simulink model "Tega0x2DNew"  (R2023b)
settings: Solver=VariableStepAuto  StartTime=0.0  StopTime=5  RelTol=1e-3
undefined symbols (not defined in the file): Ion, Lithium
libraries: spsSeriesRLCBranchLib x6, spsUniversalBridgeLib x2, spsThreePhaseParallelRLCLoadLib x1, spsBatteryLib x1, spsCurrentMeasurementLib x1, spsDieselMotorModel x1, spsDiodeLib x1, spsAC1AExcitationSystemLib x1, spsAC4AExcitationSystemLib x1, spsAC5AExcitationSystemLib x1, spsDC1AExcitationSystemLib x1, spsDC2AExcitationSystemLib x1
settings Model: Creator=HP  LastModifiedBy=HP

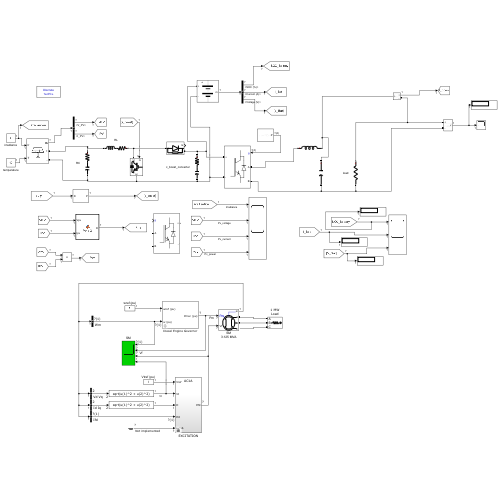
[thumbnail: Simulink's stored preview of the top-level diagram]
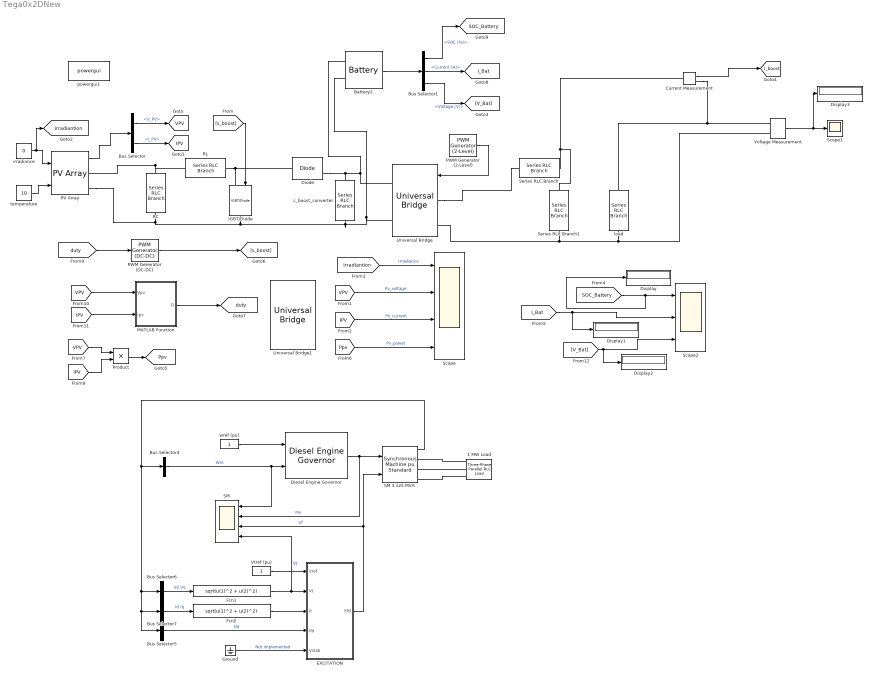
== system Tega0x2DNew ==
  1 MW Load : spsThreePhaseParallelRLCLoadLib/Three-Phase Parallel RLC Load  LConnTagsString=A|B|C  Configuration=Y (grounded)  NominalVoltage=2400  Vabc=[1e3 1e3 1e3]  Vabcp=[1e3 1e3 1e3]  NominalFrequency=60  UnbalancedPower=off  ActivePower=1e+006  InductivePower=0  CapacitivePower=0  Pabc=[10e3 9e3 11e3]  QLabc=[100 90 110]  QCabc=[100 90 110]  Pabcp=[10e3 9e3 11e3]  QLabcp=[100 90 110]  QCabcp=[100 90 110]  Measurements=None  LoadType=constant Z
  Battery2 : spsBatteryLib/Battery  BatType=Lithium-Ion  ShowTempParam=off  ThermalPreset=no  ShowAgeParam=off  NomV=12  NomQ=100  SOC=45  Batt_Tr=1  PresetModel=on  MaxQ=100  MinV=9  FullV=13.9678  Dis_rate=43.4783  R=0.0012  Normal_OP=90.4348  expZone="[12.9646      4.91304]"  current=[6.5 13 32.5]  Units=Time  Tci=20  NomT=20  T2=-30  MaxQ2=4.8  FullV2=7.1  Normal_OP2=5.655  expZone2="[6.58           1]"  Rca=0.6  ti=2000  Dp=0  Neq0=0  Tsim=1e6  Ta1=25  Qeol=5.4*0.9  Reol=0.013333*1.2  Char_age=[2.3478, 3]  Dis_age=[2.3478, 10]  N1=1500  N2=10500  N3=1000  N4=1400  Ta2=45  N5=950
  Bus Selector : BusSelector  OutputSignals=V_PV,I_PV
  Bus Selector1 : BusSelector  OutputSignals=SOC (%),Current (A),Voltage (V)
  Bus Selector4 : BusSelector  OutputSignals="Mechanical.Rotor speed  wm  (pu)"  OutputAsBus=on
  Bus Selector5 : BusSelector  OutputSignals="dq0 components.Field current  ifd (pu)"  OutputAsBus=on
  Bus Selector6 : BusSelector  OutputSignals="dq0 components.Stator voltage  vd (pu),dq0 components.Stator voltage  vq (pu)"  OutputAsBus=on
  Bus Selector7 : BusSelector  OutputSignals="dq0 components.Stator current  id (pu),dq0 components.Stator current  iq (pu)"  OutputAsBus=on
  Current Measurement : spsCurrentMeasurementLib/Current Measurement  PhasorSimulation=off  OutputType=Complex  PSBequivalent=0
  Diesel Engine Governor : spsDieselMotorModel/Diesel Engine Governor  K=40  Tr=[0.01 0.02 0.2]  Ta=[0.25 0.009 0.0384]  Tlim=[0 1.1]  Td=0.024  Pm0=0
  Diode : spsDiodeLib/Diode  Ron=0.001  Lon=0  Vf=0.8  IC=0  UseSnubber=0  Rs=500  Cs=250e-9  Measurements=on
  Display{,1..3} (4 alike) : Display
  EXCITATION : Subsystem  Variant=on  VariantControlMode=label  LabelModeActiveChoice=Variant1
      settings: AttributesFormatString=%<BlockChoice>
  Fcn1 : Fcn  Expr=sqrt(u(1)^2 + u(2)^2)
  Fcn2 : Fcn  Expr=sqrt(u(1)^2 + u(2)^2)
  Ground : Ground
  IGBT/Diode : spsIGBTDiodeLib/IGBT//Diode  Ron=1e-3  Rs=1e5  Cs=inf  Measurements=off
  MATLAB Function : MATLAB Function  TreatAsAtomicUnit=on
  PV Array : spsPVArrayLib/PV Array  Npar=6  Nser=2  PlotType=array @ 1000 W/m2 & specified temperatures  S_vec="[ 1000  500  100 ]"  Temp_C_vec="[ 45 25  ]"  ModuleName=User-defined  PlotWhenSelected=off  Pm=380.16  Ncell=72  Voc=48.7  Isc=9.98  Vm=39.6  Im=9.6  beta_Voc_pc=-0.32  alpha_Isc_pc=0.05  beta_Voc=-0.15584  alpha_Isc=0.00499  IL=10.0548  I0=7.7106e-11  nI=1.0287  Rsh=2826.5806  Rs=0.35496  RobustModel=off  RobustCellTemperature=313.3991  BAL=on  Tc=1e-6  Tfilter=5e-5
  PWM Generator (2-Level) : spsPWMGenerator2LevelLib/PWM Generator (2-Level)  ModulatorType=Single-phase full-bridge (4 pulses)  ModulatorMode=Unsynchronized  Fc=27*60  Pc=90  nF=27  MinMax="[ -1  1 ]"  SamplingTechnique=Natural  ModulatingSignals=on  m=0.8  Freq=60  Phase=0  Ts=0  ShowCarrierOutport=off
  PWM Generator (DC-DC) : spsPWMGeneratorDCDCLib/PWM Generator (DC-DC)  Fsw=5000  Ts=10e-6
  Product : Product
  RC : spsSeriesRLCBranchLib/Series RLC Branch  LConnTagsString=__new0  RConnTagsString=__new0  BranchType=RC  Resistance=1e-4  Inductance=1e-3  SetiL0=off  InitialCurrent=0  Capacitance=100e-6  Setx0=off  InitialVoltage=0  Measurements=None
  RL : spsSeriesRLCBranchLib/Series RLC Branch  LConnTagsString=__new0  RConnTagsString=__new0  BranchType=RL  Resistance=0.1  Inductance=5e-3  SetiL0=off  InitialCurrent=0  Capacitance=100e-6  Setx0=off  InitialVoltage=0  Measurements=None
  SM : Scope  NumInputPorts=4
  SM 3.125 MVA : spsSynchronousMachinepuStandardLib/Synchronous Machine pu Standard  PresetModel=No  MechanicalLoad=Mechanical power Pm  ShowDetailedParameters=on  RotorType=Salient-pole  Units=per unit standard parameters  MeasurementBus=off  NominalParameters="[ 3.125e6  2400  60]"  Reactances1=[ 31 32 33 34 35 36 37 ]  Reactances2=[ 1.56, 0.296, 0.177, 1.06, 0.177, 0.052 ]  dAxisTimeConstants=Short-circuit  qAxisTimeConstants=Open-circuit  TimeConstants1=[]  TimeConstants2=[]  TimeConstants3=[]  TimeConstants4=[]  TimeConstants5=[ 3.7, 0.05, 0.05 ]  TimeConstants6=[ 8.0, 0.03, 0.3371, 0.0295 ]  TimeConstants7=[0.024 0.006 0.006]  TimeConstants8=[]  StatorResistance=0.0036  Mechanical="[ 1.07  0 2]"  PolePairs=2  InitialConditions=[0 0 0 0 0 0 0 0 1]  SetSaturation=off  Saturation=[0.211 0.418 1.0 1.25 1.72 3.35 ;0.25 0.50 1.0 1.1 1.2 1.4]  LoadFlowParameters=[1 0 0 0]  TsPowergui=0  TsBlock=-1  IterativeModel=Trapezoidal non iterative  IterativeDiscreteModel=Trapezoidal non iterative  BusType=PV  Pref=0  Qref=0  Qmin=-Inf  Qmax=Inf  PLF=0  QLF=0
  Scope : Scope  NumInputPorts=4
  Scope1 : Scope
  Scope2 : Scope  NumInputPorts=3
  Series RLC Branch : spsSeriesRLCBranchLib/Series RLC Branch  LConnTagsString=__new0  RConnTagsString=__new0  BranchType=L  Resistance=1  Inductance=0.02  SetiL0=off  InitialCurrent=0  Capacitance=1e-6  Setx0=off  InitialVoltage=0  Measurements=None
  Series RLC Branch1 : spsSeriesRLCBranchLib/Series RLC Branch  LConnTagsString=__new0  RConnTagsString=__new0  BranchType=C  Resistance=1  Inductance=1e-3  SetiL0=off  InitialCurrent=0  Capacitance=0.006  Setx0=off  InitialVoltage=0  Measurements=None
  Universal Bridge : spsUniversalBridgeLib/Universal Bridge  Arms=2  SnubberResistance=1e5  SnubberCapacitance=inf  Device=IGBT / Diodes  Ron=1e-3  Lon=0  ForwardVoltages="[  0  0  ]"  ForwardVoltage=0  GTOparameters=[ 10e-6 , 20e-6 ]  IGBTparameters=[ 1e-6 , 2e-6 ]  Measurements=None  Measurements_2=None  converterType=Rectifier
  Universal Bridge1 : spsUniversalBridgeLib/Universal Bridge  Arms=2  SnubberResistance=1e5  SnubberCapacitance=inf  Device=IGBT / Diodes  Ron=1e-3  Lon=0  ForwardVoltages="[  0  0  ]"  ForwardVoltage=0  GTOparameters=[ 10e-6 , 20e-6 ]  IGBTparameters=[ 1e-6 , 2e-6 ]  Measurements=None  Measurements_2=None  converterType=Rectifier
  Voltage Measurement : spsVoltageMeasurementLib/Voltage Measurement  PhasorSimulation=off  OutputType=Complex  PSBequivalent=0
  "Vtref (pu) " : Constant
  c_boost_converter : spsSeriesRLCBranchLib/Series RLC Branch  LConnTagsString=__new0  RConnTagsString=__new0  BranchType=RC  Resistance=1e-4  Inductance=1e-3  SetiL0=off  InitialCurrent=0  Capacitance=3300e-6  Setx0=off  InitialVoltage=0  Measurements=None
  irradiance : Constant  Value=0
  load : spsSeriesRLCBranchLib/Series RLC Branch  LConnTagsString=__new0  RConnTagsString=__new0  BranchType=R  Resistance=10  Inductance=1e-3  SetiL0=off  InitialCurrent=0  Capacitance=3300e-6  Setx0=off  InitialVoltage=0  Measurements=None
  powergui1 : spspowerguiLib/powergui  Priority=1  SimulationMode=Discrete  SampleTime=1e-05  frequency=60  Iterations=50  frequencyindice=0  Pbase=100e6  ErrMax=1e-4  UnitsV=kV  UnitsW=MW  buscounter=0  FunctionMessages=off  echomessages=off  EnableUseOfTLC=off  CurrentSourceSwitches=off  DisableSnubberDevices=off  DisableRonSwitches=off  DisableVfSwitches=off  DisplayEquations=off  AutomaticDiscreteSolvers=off  SolverType=Tustin/Backward Euler (TBE)  Interpol=off  ExternalGateDelay=off  methode=off  Ts=100  x0status=blocks  SPID=on  SwTol=0  HookPort=off  NonlinearTolerance=1e-4  nMaxIteration=100  ContinueOnMaxIteration=off  RestoreLinks=warning  ResistiveCurrentMeasurement=off  Frange=[0:2:500]  Ylog=off  Xlog=on  ShowGrid=off  save=off  variable=ZData  structure=0  ZoomFFT=off  StartTime=0.0  cycles=1  DisplayStyle=1  fundamental=60  FreqAxis=off  MaxFrequency=1000  frequencyindicesteady=1  RmsSteady=1  display=off
  temperature : Constant  Value=10
  wref (pu) : Constant
  tag scope: IPV=global, I_Bat=global, I_boost=global, Ppv=global, SOC_Battery=global, VPV=global, duty=global, irradiantion=global
  wires:
  PV Array/1 -> Bus Selector/1
  Bus Selector/1 -> [VPV]  "<V_PV>"
  Bus Selector/2 -> [IPV]  "<I_PV>"
  temperature/1 -> PV Array/2
  irradiance/1 -> [irradiantion], PV Array/1
  [s_boost] -> IGBT/Diode/1
  Voltage Measurement/1 -> Display3/1, Scope1/1
  Current Measurement/1 -> [I_boost]
  [irradiantion] -> Scope/1  "Irradiance"
  [VPV] -> Scope/2  "Pv_voltage"
  [IPV] -> Scope/3  "Pv_current"
  Product/1 -> [Ppv]
  [VPV] -> Product/1
  [IPV] -> Product/2
  PWM Generator (DC-DC)/1 -> [s_boost]
  [duty] -> PWM Generator (DC-DC)/1
  [VPV] -> MATLAB Function/1(Vpv)
  [IPV] -> MATLAB Function/2(Ipv)
  MATLAB Function/1(D) -> [duty]
  PWM Generator (2-Level)/1 -> Universal Bridge/1
  [Ppv] -> Scope/4  "Pv_power"
  Battery2/1 -> Bus Selector1/1
  Bus Selector1/1 -> [SOC_Battery]  "<SOC (%)>"
  Bus Selector1/2 -> [I_Bat]  "<Current (A)>"
  Bus Selector1/3 -> [V_Bat]  "<Voltage (V)>"
  [I_Bat] -> Display1/1, Scope2/2
  [V_Bat] -> Display2/1, Scope2/3
  [SOC_Battery] -> Display/1, Scope2/1
  SM 3.125 MVA/1 -> Bus Selector4/1, Bus Selector6/1, Bus Selector7/1, Bus Selector5/1
  Fcn1/1 -> SM/4, EXCITATION/2(Vt)  "Vt"
  EXCITATION/1(Efd) -> SM/3, SM 3.125 MVA/2  "Vf"
  wref (pu)/1 -> Diesel Engine Governor/1
  Bus Selector5/1 -> EXCITATION/4(Ifd)  "Ifd"
  Diesel Engine Governor/1 -> SM/2, SM 3.125 MVA/1  "Pm"
  "Vtref (pu) "/1 -> EXCITATION/1(Vref)
  Bus Selector7/1 -> Fcn2/1  "Id Iq"
  Ground/1 -> EXCITATION/5(Vstab)  "Not implemented"
  Bus Selector6/1 -> Fcn1/1  "Vd Vq"
  Fcn2/1 -> EXCITATION/3(It)
  Bus Selector4/1 -> Diesel Engine Governor/2, SM/1  "Wm"
  connections:
  RC/LConn1 -- RL/RConn1 -- PV Array/RConn1
  RC/RConn1 -- PV Array/RConn2 -- Battery2/LConn2 -- Universal Bridge/RConn2 -- c_boost_converter/RConn1 -- IGBT/Diode/RConn1
  RL/LConn1 -- Diode/LConn1 -- IGBT/Diode/LConn1
  Diode/RConn1 -- Battery2/LConn1 -- Universal Bridge/RConn1 -- c_boost_converter/LConn1
  Universal Bridge/LConn1 -- Series RLC Branch/LConn1
  Series RLC Branch1/RConn1 -- Voltage Measurement/LConn2 -- load/RConn1 -- Universal Bridge/LConn2
  Voltage Measurement/LConn1 -- load/LConn1 -- Current Measurement/RConn1
  Current Measurement/LConn1 -- Series RLC Branch1/LConn1 -- Series RLC Branch/RConn1
  1 MW Load/LConn2 -- SM 3.125 MVA/RConn2
  1 MW Load/LConn3 -- SM 3.125 MVA/RConn3
  1 MW Load/LConn1 -- SM 3.125 MVA/RConn1

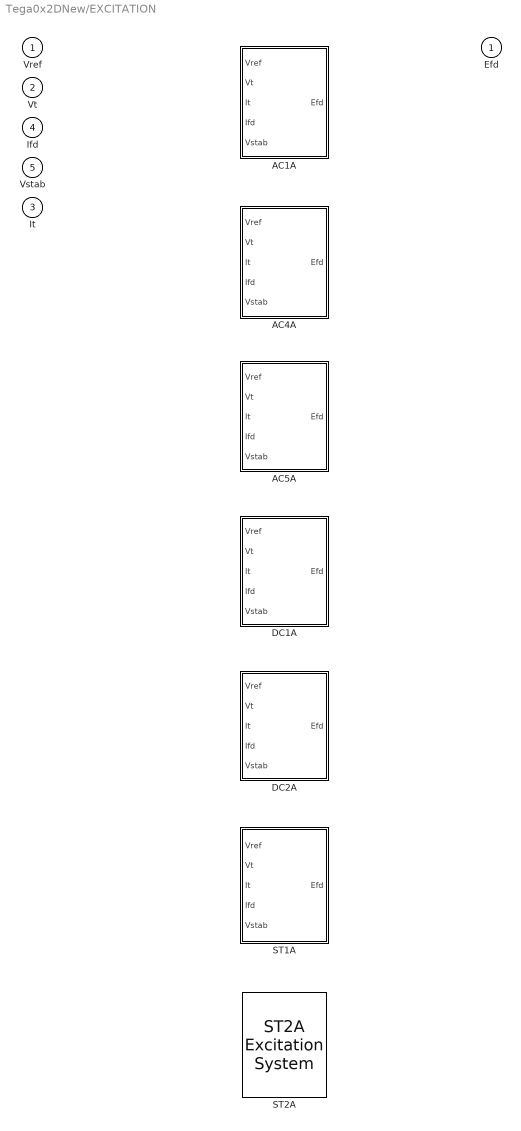
== system Tega0x2DNew/EXCITATION ==
  Vref : Inport
  Vt : Inport  Port=2
  It : Inport  Port=3
  Ifd : Inport  Port=4
  Vstab : Inport  Port=5
  AC1A : Subsystem  VariantControl=Variant1
  AC4A : Subsystem  VariantControl=Variant2
  AC5A : Subsystem  VariantControl=Variant3
  DC1A : Subsystem  VariantControl=Variant4
  DC2A : Subsystem  VariantControl=Variant5
  ST1A : Subsystem  VariantControl=Variant6
  ST2A : spsST2AExcitationSystemLib/ST2A Excitation System  VariantControl=Variant7  Tr=20e-3  KaTa=[120 0.15]  VRminmax=[0 1.0]  KfTf=[0.05 1.0]  KeTe=[1.0 0.5]  KI=8.0  Kp=4.88  Xd=1.56  Kc=1.82  v0=[1,1.42734]  I0=0.2739  TsBlock=-2
  Efd : Outport  VectorParamsAs1DForOutWhenUnconnected=off

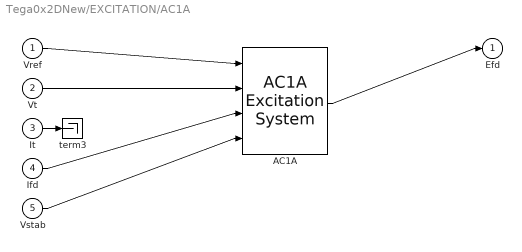
== system Tega0x2DNew/EXCITATION/AC1A ==
  Vref : Inport
  Vt : Inport  Port=2
  It : Inport  Port=3
  Ifd : Inport  Port=4
  Vstab : Inport  Port=5
  AC1A : spsAC1AExcitationSystemLib/AC1A Excitation System  Tr=20e-3  KaTa=[400 0.02]  VAminmax=[-14.5 14.5]  VRminmax=[-5.43 6.03]  KfTf=[0.03 1.0]  TbTc=[0 0]  KeTe=[1.0 0.80]  Ve12=[4.18 3.14]  SeVe12=[0.10 0.03]  Kd=0.38  Kc=0.20  v0=[1 1.4273]  TsBlock=-2
  term3 : Terminator
  Efd : Outport  VectorParamsAs1DForOutWhenUnconnected=off
  wires:
  It/1 -> term3/1
  AC1A/1 -> Efd/1
  Vstab/1 -> AC1A/4
  Ifd/1 -> AC1A/3
  Vt/1 -> AC1A/2
  Vref/1 -> AC1A/1

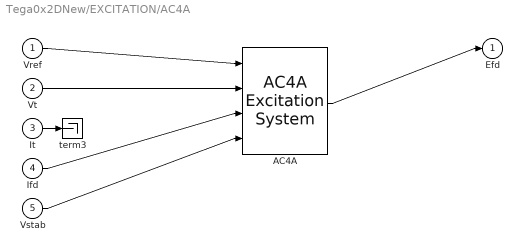
== system Tega0x2DNew/EXCITATION/AC4A ==
  Vref : Inport
  Vt : Inport  Port=2
  It : Inport  Port=3
  Ifd : Inport  Port=4
  Vstab : Inport  Port=5
  AC4A : spsAC4AExcitationSystemLib/AC4A Excitation System  Tr=20e-3  KaTa=[200 0.015]  VIminmax=[-10 10]  VRminmax=[-4.53 5.64]  TbTc=[10 1.0]  Kc=0  v0=[1,1.42734]  TsBlock=-2
  term3 : Terminator
  Efd : Outport  VectorParamsAs1DForOutWhenUnconnected=off
  wires:
  It/1 -> term3/1
  AC4A/1 -> Efd/1
  Vstab/1 -> AC4A/4
  Ifd/1 -> AC4A/3
  Vt/1 -> AC4A/2
  Vref/1 -> AC4A/1

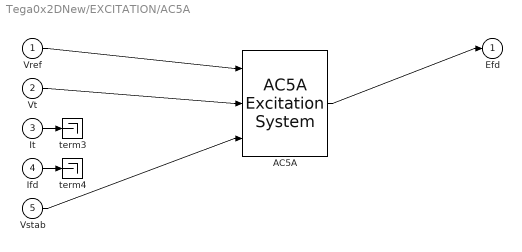
== system Tega0x2DNew/EXCITATION/AC5A ==
  Vref : Inport
  Vt : Inport  Port=2
  It : Inport  Port=3
  Ifd : Inport  Port=4
  Vstab : Inport  Port=5
  AC5A : spsAC5AExcitationSystemLib/AC5A Excitation System  Tr=20e-3  KaTa=[100 0.02]  VRminmax=[-7.3 7.3]  KfTf=[0.03 1 0 0]  KeTe=[1.0 0.02]  Efd12=[5.6 0.75*5.6]  SeEfd12=[0.86 0.5]  v0=[1,1.42734]  TsBlock=-2
  term3 : Terminator
  term4 : Terminator
  Efd : Outport  VectorParamsAs1DForOutWhenUnconnected=off
  wires:
  Ifd/1 -> term4/1
  It/1 -> term3/1
  AC5A/1 -> Efd/1
  Vstab/1 -> AC5A/3
  Vt/1 -> AC5A/2
  Vref/1 -> AC5A/1

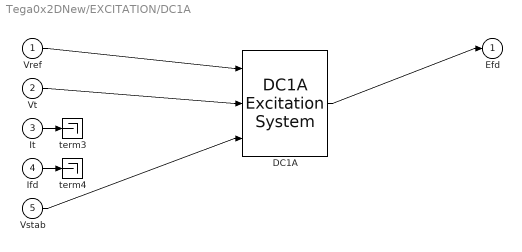
== system Tega0x2DNew/EXCITATION/DC1A ==
  Vref : Inport
  Vt : Inport  Port=2
  It : Inport  Port=3
  Ifd : Inport  Port=4
  Vstab : Inport  Port=5
  DC1A : spsDC1AExcitationSystemLib/DC1A Excitation System  Tr=20e-3  KaTa=[46 0.06]  VRminmax=[-0.9 1.0]  KfTf=[0.05 1.5]  TbTc=[0 0]  KeTe=[0.05 0.46]  Efd12=[3.1 2.3]  SeEfd12=[0.33 0.10]  v0=[1,1.42734]  TsBlock=-2
  term3 : Terminator
  term4 : Terminator
  Efd : Outport  VectorParamsAs1DForOutWhenUnconnected=off
  wires:
  Ifd/1 -> term4/1
  It/1 -> term3/1
  DC1A/1 -> Efd/1
  Vstab/1 -> DC1A/3
  Vt/1 -> DC1A/2
  Vref/1 -> DC1A/1

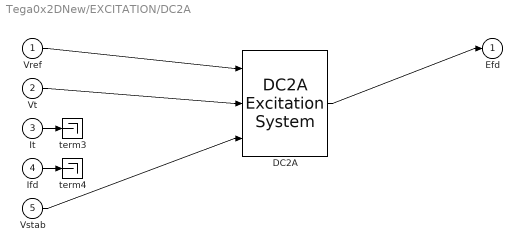
== system Tega0x2DNew/EXCITATION/DC2A ==
  Vref : Inport
  Vt : Inport  Port=2
  It : Inport  Port=3
  Ifd : Inport  Port=4
  Vstab : Inport  Port=5
  DC2A : spsDC2AExcitationSystemLib/DC2A Excitation System  Tr=20e-3  KaTa=[46 0.06]  VRminmax=[-4.9 4.95]  KfTf=[0.05 1.5]  TbTc=[0 0]  KeTe=[0.05 0.46]  Efd12=[3.05 2.29]  SeEfd12=[0.279 0.117]  v0=[1,1.42734]  TsBlock=-2
  term3 : Terminator
  term4 : Terminator
  Efd : Outport  VectorParamsAs1DForOutWhenUnconnected=off
  wires:
  Ifd/1 -> term4/1
  It/1 -> term3/1
  DC2A/1 -> Efd/1
  Vstab/1 -> DC2A/3
  Vt/1 -> DC2A/2
  Vref/1 -> DC2A/1

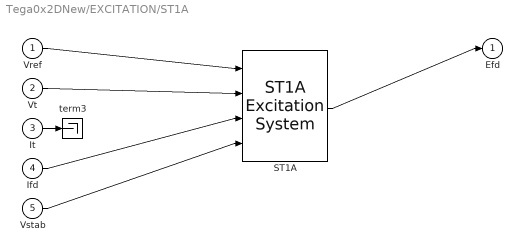
== system Tega0x2DNew/EXCITATION/ST1A ==
  Vref : Inport
  Vt : Inport  Port=2
  It : Inport  Port=3
  Ifd : Inport  Port=4
  Vstab : Inport  Port=5
  ST1A : spsST1AExcitationSystemLib/ST1A Excitation System  Tr=20e-3  KaTa=[210 0.001]  VIminmax=[-999 999]  VAminmax=[-999 999]  VRminmax=[-6.0 6.43]  KfTf=[0.001 1]  TbTc=[0 0 0 0]  KLR=1  ILR=2  Kc=0.038  v0=[1,1.42734]  TsBlock=-2
  term3 : Terminator
  Efd : Outport  VectorParamsAs1DForOutWhenUnconnected=off
  wires:
  It/1 -> term3/1
  ST1A/1 -> Efd/1
  Vstab/1 -> ST1A/4
  Ifd/1 -> ST1A/3
  Vt/1 -> ST1A/2
  Vref/1 -> ST1A/1

== matlab function Tega0x2DNew/MATLAB Function ==
  data: Vpv input; D output; Ipv input
function D = PandO(Vpv, Ipv)

persistent Dprev Pprev Vprev

if isempty(Dprev)
    Dprev = 0.7;
    Vprev = 190;
    Pprev = 2000;
end

deltaD = 125e-6;

%calculate measured aerray power
Ppv = Vpv*Ipv; 

%Increase or decrease duty cycle based on conditions
if (Ppv-Pprev) ~= 0
    if (Ppv-Pprev) > 0
        if (Vpv-Vprev) > 0
            D = Dprev - deltaD;
        else
            D = Dprev + deltaD;
        end
    else
        if (Vpv-Vprev) > 0
            D = Dprev + deltaD;
        else
            D = Dprev - deltaD;
        end
    end
else
    D =Dprev;
end

%Update internal values
Dprev = D;
Vprev = Vpv;
Pprev = Ppv;
